simulink model "nonlinearSim"  (R2016a)
settings: Solver=ode45  StartTime=0.0  StopTime=20  MaxStep=1e-3  RelTol=1e-3
values from neighbouring files (symbols this model uses):
  Taction = .1    (= 0.1)    [simFullOrderModel.m]    (also in simReducedOrderController.m = 2)
  x0 = [0 0 0 0]'    [simFullOrderModel.m]    (also in simReducedOrderController.m = H*x0)
undefined symbols (not defined in the file or in its folder): tStar, uStar, xStar
libraries: simulink x1
settings Model: Creator=xingye  LastModifiedBy=xingye

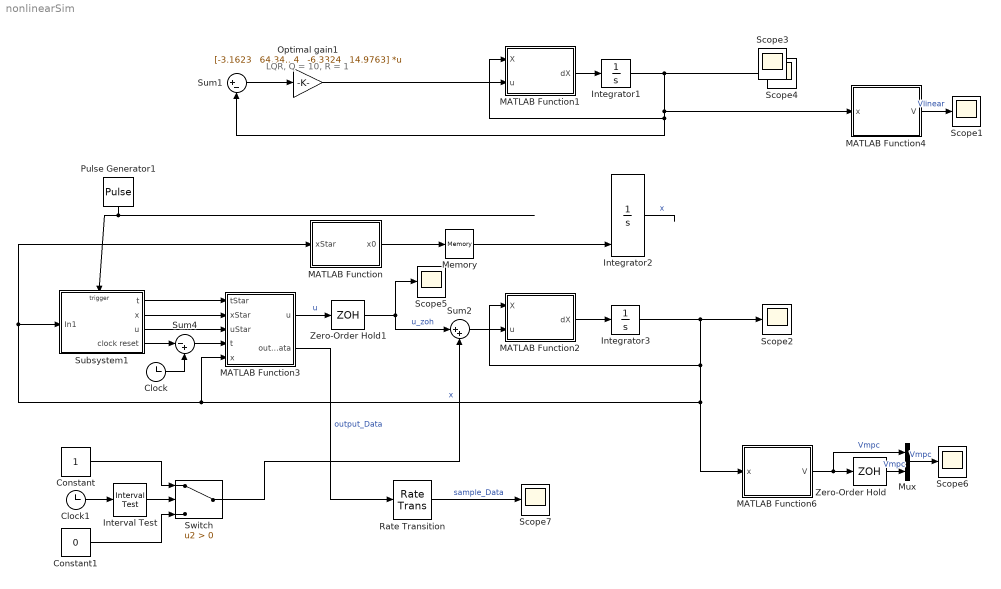
== system nonlinearSim ==
  note: LQR, Q = 10, R = 1
  Clock : Clock
  Clock1 : Clock
  Constant : Constant
  Constant1 : Constant  Value=0
  Integrator1 : Integrator  InitialCondition=x0
  Integrator2 : Integrator  ExternalReset=rising  InitialConditionSource=external  InitialCondition=x0
  Integrator3 : Integrator  InitialCondition=x0
  Interval Test : simulink/Logic and Bit Operations/Interval Test  IntervalClosedRight=on  uplimit=12  IntervalClosedLeft=on  lowlimit=11.5  OutDataTypeStr=boolean
  MATLAB Function : MATLAB Function  TreatAsAtomicUnit=on
  MATLAB Function1 : MATLAB Function  TreatAsAtomicUnit=on
  MATLAB Function2 : MATLAB Function  TreatAsAtomicUnit=on
  MATLAB Function3 : MATLAB Function  TreatAsAtomicUnit=on
  MATLAB Function4 : MATLAB Function  TreatAsAtomicUnit=on
  MATLAB Function6 : MATLAB Function  TreatAsAtomicUnit=on
  Memory : Memory  X0=x0
  Mux : Mux  Inputs=2
  Optimal gain1 : Gain  Gain="[-3.1623   64.3424   -6.3324   14.9763]"  Multiplication=Matrix(K*u)
  Pulse Generator1 : DiscretePulseGenerator  PulseType=Time based  Period=Taction  PulseWidth=50
  Rate Transition : RateTransition  OutPortSampleTime=2
  Scope{1..7} (7 alike) : Scope
  Subsystem1 : Subsystem
  Sum1 : Sum  Inputs=|+-
  Sum2 : Sum  Inputs=|++
  Sum4 : Sum  Inputs=|-+
  Switch : Switch  Criteria=u2 > Threshold
  Zero-Order Hold : ZeroOrderHold  SampleTime=Taction
  Zero-Order Hold1 : ZeroOrderHold  SampleTime=Taction
  wires:
  MATLAB Function1/1(dX) -> Integrator1/1
  Sum1/1 -> Optimal gain1/1
  Optimal gain1/1 -> MATLAB Function1/2(u)
  Pulse Generator1/1 -> Subsystem1/Trigger
  Subsystem1/1(t) -> MATLAB Function3/1(tStar)
  Sum4/1 -> MATLAB Function3/4(t)
  Clock/1 -> Sum4/2
  Subsystem1/4(clock reset) -> Sum4/1
  Subsystem1/2(x) -> MATLAB Function3/2(xStar)
  MATLAB Function3/1(u) -> Zero-Order Hold1/1  "u"
  Mux/1 -> Scope6/1  "Vmpc"
  Integrator1/1 -> MATLAB Function4/1(x), Sum1/2, MATLAB Function1/1(X), Scope4/1
  MATLAB Function4/1(V) -> Scope1/1  "Vlinear"
  MATLAB Function6/1(V) -> Mux/1, Zero-Order Hold/1  "Vmpc"
  Zero-Order Hold/1 -> Mux/2  "Vmpc"
  Sum2/1 -> MATLAB Function2/2(u)
  Constant/1 -> Switch/1
  Switch/1 -> Sum2/2
  Interval Test/1 -> Switch/2
  Clock1/1 -> Interval Test/1
  Constant1/1 -> Switch/3
  Zero-Order Hold1/1 -> Sum2/1, Scope5/1  "u_zoh"
  Subsystem1/3(u) -> MATLAB Function3/3(uStar)
  MATLAB Function2/1(dX) -> Integrator3/1
  Integrator3/1 -> Scope2/1, MATLAB Function2/1(X), MATLAB Function/1(xStar), Subsystem1/1(In1), MATLAB Function3/5(x), MATLAB Function6/1(x)  "x"
  MATLAB Function/1(x0) -> Memory/1
  Memory/1 -> Integrator2/3
  MATLAB Function3/2(output_Data) -> Rate Transition/1  "output_Data"
  Integrator2/1 -> ?  "x"
  Rate Transition/1 -> Scope7/1  "sample_Data"

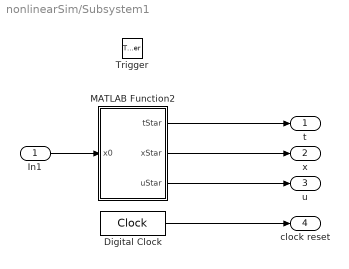
== system nonlinearSim/Subsystem1 ==
  In1 : Inport
  Trigger : TriggerPort  VariantControl=Variant  PortDimensions=1
  Digital Clock : DigitalClock  SampleTime=-1
  MATLAB Function2 : MATLAB Function  TreatAsAtomicUnit=on
  t : Outport  InitialOutput=tStar
  x : Outport  Port=2  InitialOutput=xStar
  u : Outport  Port=3  InitialOutput=uStar
  clock reset : Outport  Port=4  InitialOutput=0
  wires:
  MATLAB Function2/1(tStar) -> t/1
  In1/1 -> MATLAB Function2/1("x0 ")
  Digital Clock/1 -> clock reset/1
  MATLAB Function2/2(xStar) -> x/1
  MATLAB Function2/3(uStar) -> u/1

== matlab function nonlinearSim/MATLAB Function1 ==
  data: X input; u input; dX output
function dX = fcn(X, u)
%#codegen

x = X(1:2) + [0 pi/2]';
xdot = X(3:4);

M = ([[2,-sin(x(2,:))/2];[-sin(x(2,:))/2,1/3]]);
f = ([[u(:,1)+(xdot(2,:)^2*cos(x(2,:)))/2];[-(981*cos(x(2,:)))/200]]);

xddot = M\f;

dX = [xdot; xddot];

== matlab function nonlinearSim/MATLAB Function4 ==
  data: x input; V output size=1
function V = LyapunovFunction(x)
	%#codegen
	
	
	x = reshape(x, 4, 1);
	P = [
		17.8236  -33.7375   10.7063   -8.4552
		-33.7375  183.9190  -48.9624   41.6848
		10.7063  -48.9624   14.9440  -12.0628
		-8.4552   41.6848  -12.0628   10.6193
		];	% Q = 10, R = 1
	
	V = x'* P* x;

== matlab function nonlinearSim/MATLAB Function2 ==
  data: X input; u input; dX output
function dX = fcn(X, u)
%#codegen

x = X(1:2) + [0 pi/2]';
xdot = X(3:4);

M = ([[2,-sin(x(2,:))/2];[-sin(x(2,:))/2,1/3]]);
f = ([[u(:,1)+(xdot(2,:)^2*cos(x(2,:)))/2];[-(981*cos(x(2,:)))/200]]);

xddot = M\f;

dX = [xdot; xddot];

== matlab function nonlinearSim/MATLAB Function3 ==
  data: tStar input; xStar input; uStar input; u output; t input; x input; output_Data output
function [u, output_Data] = interp_u(tStar, xStar, uStar, t, x)
%#codegen


u = interp1(tStar, uStar, t,'linear');	% better for the accuracy
% u = interp1(tStar, uStar, t,'spline');

% P = [
% 	17.8236  -33.7375   10.7063   -8.4552
% 	-33.7375  183.9190  -48.9624   41.6848
% 	10.7063  -48.9624   14.9440  -12.0628
% 	-8.4552   41.6848  -12.0628   10.6193
% 	];	% Q = 10, R = 1

P = [
	  0.04         -0.11          0.03         -0.03
	 -0.11          0.94         -0.12          0.18
	  0.03         -0.12          0.03         -0.03
	 -0.03          0.18         -0.03          0.04
	];% J(x)

output_Data = x'* P* x;

== matlab function nonlinearSim/Subsystem1/MATLAB Function2 ==
  data: tStar output; x0 input; xStar output; uStar output
function [tStar, xStar, uStar] = fcn(x0)
%#codegen
coder.extrinsic('funEquilibrium');
nNodes = 120 + 1;
% nNodes = 12000 + 1;
tStar = zeros(nNodes,1);
xStar = zeros(nNodes,4);
uStar = zeros(nNodes,1);


L = zeros(2);
% L = [pi/15 pi/15; 0 0];
% L = [0.1744 0.0437; 0.2531 0.0624];
H = [1 0 0 0; L(1,1) 0 L(1,2) 0; 0 0 1 0; L(2,1) 0 L(2,2) 0];
% x0 = H*x0;

[~, ~, tStar, xStar, uStar] = funEquilibrium(x0, nNodes, L);

== matlab function nonlinearSim/MATLAB Function ==
  data: xStar input; x0 output
function x0 = fcn(xStar)
%#codegen

% H = eye(4);
% H = [1 0 0 0; pi/6 0 0 0; 0 0 1 0; 0 0 pi/6 0];
% H = [1 0 0 0; 0 0 0 0; 0 0 1 0; 0 0 0 0];
H = [1 0 0 0; 0.1744 0 0.0437 0; 0 0 1 0; 0.2531 0 0.0624 0];
x0 = H*xStar;

== matlab function nonlinearSim/MATLAB Function6 ==
  data: x input; V output size=1
function V = LyapunovFunction(x)
	%#codegen
	
	
	x = reshape(x, 4, 1);
	P = [
		17.8236  -33.7375   10.7063   -8.4552
		-33.7375  183.9190  -48.9624   41.6848
		10.7063  -48.9624   14.9440  -12.0628
		-8.4552   41.6848  -12.0628   10.6193
		];	% Q = 10, R = 1
	
	V = x'* P* x;
